simulink model "MdXX_RspOutComm1"  (R2018b)
settings: Solver=FixedStepDiscrete  StartTime=0.0  StopTime=10.0  FixedStep=0.01  RelTol=1e-3
undefined symbols (not defined in the file or in its folder): KeSMSuRspStatHldTm_Val, MdRspLocal2, SrcReqTp1
libraries: simulink x64, RspLib x32
(part 3 of 4)

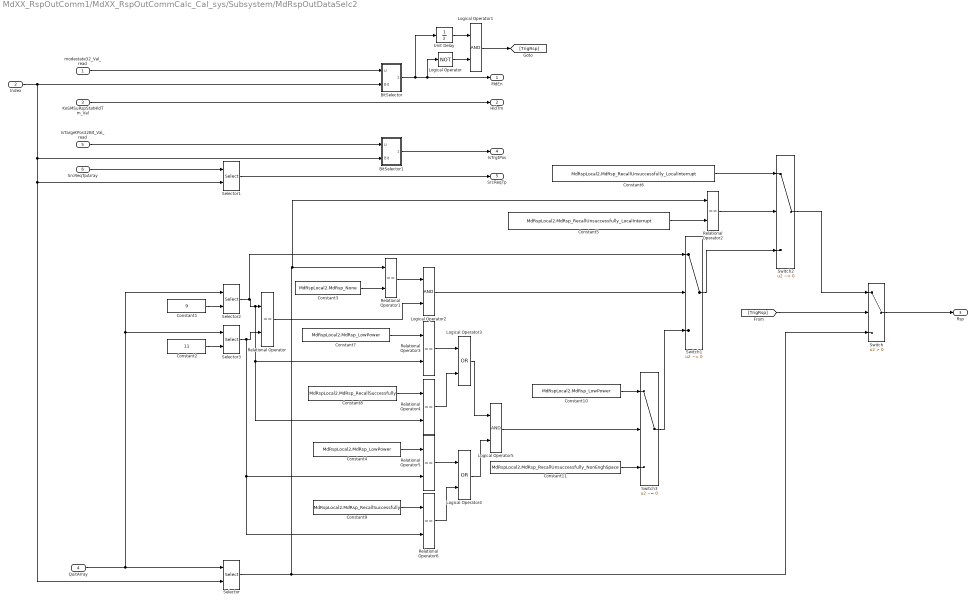
== system MdXX_RspOutComm1/MdXX_RspOutCommCalc_Cal_sys/Subsystem/MdRspOutDataSelc2 ==
  modestate32_Val_read : Inport
  Index : Inport  Port=2
  KeSMSuRspStatHldTm_Val : Inport  Port=3
  QuitArray : Inport  Port=4
  IsTargetPos32Bit_Val_read : Inport  Port=5
  SrcReqTpArray : Inport  Port=6
  BitSelector : Subsystem
  BitSelector1 : Subsystem
  Constant1 : Constant  Value=9  OutDataTypeStr=uint8
  Constant10 : Constant  Value=MdRspLocal2.MdRsp_LowPower  OutDataTypeStr=Enum: MdRspLocal2
  Constant11 : Constant  Value=MdRspLocal2.MdRsp_RecallUnsuccessfully_NonEnghSpace  OutDataTypeStr=Enum: MdRspLocal2
  Constant2 : Constant  Value=11  OutDataTypeStr=uint8
  Constant3 : Constant  Value=MdRspLocal2.MdRsp_None  OutDataTypeStr=Enum: MdRspLocal2
  Constant4 : Constant  Value=MdRspLocal2.MdRsp_LowPower  OutDataTypeStr=Enum: MdRspLocal2
  Constant5 : Constant  Value=MdRspLocal2.MdRsp_RecallUnsuccessfully_LocalInterrupt  OutDataTypeStr=Enum: MdRspLocal2
  Constant6 : Constant  Value=MdRspLocal2.MdRsp_RecallUnsuccessfully_LocalInterrupt  OutDataTypeStr=Enum: MdRspLocal2
  Constant7 : Constant  Value=MdRspLocal2.MdRsp_LowPower  OutDataTypeStr=Enum: MdRspLocal2
  Constant8 : Constant  Value=MdRspLocal2.MdRsp_RecallSuccessfully  OutDataTypeStr=Enum: MdRspLocal2
  Constant9 : Constant  Value=MdRspLocal2.MdRsp_RecallSuccessfully  OutDataTypeStr=Enum: MdRspLocal2
  Logical Operator : Logic  Operator=NOT  AllPortsSameDT=off  OutDataTypeStr=boolean
  Logical Operator1 : Logic  AllPortsSameDT=off  OutDataTypeStr=boolean
  Logical Operator2 : Logic  AllPortsSameDT=off  OutDataTypeStr=boolean
  Logical Operator3 : Logic  Operator=OR  AllPortsSameDT=off  OutDataTypeStr=boolean
  Logical Operator4 : Logic  Operator=OR  AllPortsSameDT=off  OutDataTypeStr=boolean
  Logical Operator5 : Logic  AllPortsSameDT=off  OutDataTypeStr=boolean
  Relational Operator{,1..6} (7 alike) : RelationalOperator  Operator===  OutDataTypeStr=boolean  RndMeth=Simplest
  Selector{,1..3} (4 alike) : Selector  IndexMode=Zero-based  InputPortWidth=32  IndexOptions=Index vector (port)  Indices=[1 3]  OutputSizes=1
  Switch : Switch  Criteria=u2 > Threshold
  Switch1 : Switch  Criteria=u2 ~= 0
  Switch2 : Switch  Criteria=u2 ~= 0
  Switch3 : Switch  Criteria=u2 ~= 0
  Unit Delay : UnitDelay  SampleTime=-1
  MdEn : Outport
  HldTm : Outport  Port=2
  Rsp : Outport  Port=3
  IsTrgtPos : Outport  Port=4
  SrcReqTp : Outport  Port=5
  wires:
  KeSMSuRspStatHldTm_Val/1 -> HldTm/1
  Index/1 -> BitSelector/2(Bit), Selector/2, Selector1/2, BitSelector1/2(Bit)
  Selector/1 -> Relational Operator2/1, Relational Operator1/1, Switch/3
  BitSelector/1(BitOut) -> Unit Delay/1, Logical Operator/1, MdEn/1
  modestate32_Val_read/1 -> BitSelector/1(U)
  BitSelector1/1(BitOut) -> IsTrgtPos/1
  IsTargetPos32Bit_Val_read/1 -> BitSelector1/1(U)
  QuitArray/1 -> Selector3/1, Selector2/1, Selector/1
  SrcReqTpArray/1 -> Selector1/1
  Selector1/1 -> SrcReqTp/1
  Unit Delay/1 -> Logical Operator1/1
  Logical Operator/1 -> Logical Operator1/2
  Logical Operator1/1 -> [TrigRsp]
  [TrigRsp] -> Switch/2
  Constant1/1 -> Selector2/2
  Constant2/1 -> Selector3/2
  Selector2/1 -> Switch1/1, Relational Operator/1, Relational Operator4/2, Relational Operator3/2
  Relational Operator/1 -> Logical Operator2/2
  Relational Operator1/1 -> Logical Operator2/1
  Constant3/1 -> Relational Operator1/2
  Logical Operator2/1 -> Switch1/2
  Switch/1 -> Rsp/1
  Constant5/1 -> Relational Operator2/2
  Relational Operator2/1 -> Switch2/2
  Constant6/1 -> Switch2/1
  Switch1/1 -> Switch2/3
  Switch2/1 -> Switch/1
  Switch3/1 -> Switch1/3
  Constant7/1 -> Relational Operator3/1
  Relational Operator3/1 -> Logical Operator3/1
  Relational Operator4/1 -> Logical Operator3/2
  Constant8/1 -> Relational Operator4/1
  Relational Operator5/1 -> Logical Operator4/1
  Constant4/1 -> Relational Operator5/1
  Relational Operator6/1 -> Logical Operator4/2
  Constant9/1 -> Relational Operator6/1
  Selector3/1 -> Relational Operator6/2, Relational Operator5/2, Relational Operator/2
  Logical Operator3/1 -> Logical Operator5/1
  Logical Operator4/1 -> Logical Operator5/2
  Logical Operator5/1 -> Switch3/2
  Constant10/1 -> Switch3/1
  Constant11/1 -> Switch3/3

== system MdXX_RspOutComm1/MdXX_RspOutCommCalc_Cal_sys/Subsystem/MdRspOutDataSelc20 ==
  modestate32_Val_read : Inport
  Index : Inport  Port=2
  KeSMSuRspStatHldTm_Val : Inport  Port=3
  QuitArray : Inport  Port=4
  IsTargetPos32Bit_Val_read : Inport  Port=5
  SrcReqTpArray : Inport  Port=6
  BitSelector : Subsystem
  BitSelector1 : Subsystem
  Selector : Selector  IndexMode=Zero-based  InputPortWidth=32  IndexOptions=Index vector (port)  Indices=[1 3]  OutputSizes=1
  Selector1 : Selector  IndexMode=Zero-based  InputPortWidth=32  IndexOptions=Index vector (port)  Indices=[1 3]  OutputSizes=1
  MdEn : Outport
  HldTm : Outport  Port=2
  Rsp : Outport  Port=3
  IsTrgtPos : Outport  Port=4
  SrcReqTp : Outport  Port=5
  wires:
  KeSMSuRspStatHldTm_Val/1 -> HldTm/1
  Index/1 -> BitSelector/2(Bit), Selector/2, Selector1/2, BitSelector1/2(Bit)
  Selector/1 -> Rsp/1
  BitSelector/1(BitOut) -> MdEn/1
  modestate32_Val_read/1 -> BitSelector/1(U)
  BitSelector1/1(BitOut) -> IsTrgtPos/1
  IsTargetPos32Bit_Val_read/1 -> BitSelector1/1(U)
  QuitArray/1 -> Selector/1
  SrcReqTpArray/1 -> Selector1/1
  Selector1/1 -> SrcReqTp/1

== system MdXX_RspOutComm1/MdXX_RspOutCommCalc_Cal_sys/Subsystem/MdRspOutDataSelc21 ==
  modestate32_Val_read : Inport
  Index : Inport  Port=2
  KeSMSuRspStatHldTm_Val : Inport  Port=3
  QuitArray : Inport  Port=4
  IsTargetPos32Bit_Val_read : Inport  Port=5
  SrcReqTpArray : Inport  Port=6
  BitSelector : Subsystem
  BitSelector1 : Subsystem
  Selector : Selector  IndexMode=Zero-based  InputPortWidth=32  IndexOptions=Index vector (port)  Indices=[1 3]  OutputSizes=1
  Selector1 : Selector  IndexMode=Zero-based  InputPortWidth=32  IndexOptions=Index vector (port)  Indices=[1 3]  OutputSizes=1
  MdEn : Outport
  HldTm : Outport  Port=2
  Rsp : Outport  Port=3
  IsTrgtPos : Outport  Port=4
  SrcReqTp : Outport  Port=5
  wires:
  Selector1/1 -> SrcReqTp/1
  SrcReqTpArray/1 -> Selector1/1
  QuitArray/1 -> Selector/1
  IsTargetPos32Bit_Val_read/1 -> BitSelector1/1(U)
  BitSelector1/1(BitOut) -> IsTrgtPos/1
  modestate32_Val_read/1 -> BitSelector/1(U)
  BitSelector/1(BitOut) -> MdEn/1
  Selector/1 -> Rsp/1
  Index/1 -> BitSelector1/2(Bit), Selector1/2, Selector/2, BitSelector/2(Bit)
  KeSMSuRspStatHldTm_Val/1 -> HldTm/1

== system MdXX_RspOutComm1/MdXX_RspOutCommCalc_Cal_sys/Subsystem/MdRspOutDataSelc22 ==
  modestate32_Val_read : Inport
  Index : Inport  Port=2
  KeSMSuRspStatHldTm_Val : Inport  Port=3
  QuitArray : Inport  Port=4
  IsTargetPos32Bit_Val_read : Inport  Port=5
  SrcReqTpArray : Inport  Port=6
  BitSelector : Subsystem
  BitSelector1 : Subsystem
  Selector : Selector  IndexMode=Zero-based  InputPortWidth=32  IndexOptions=Index vector (port)  Indices=[1 3]  OutputSizes=1
  Selector1 : Selector  IndexMode=Zero-based  InputPortWidth=32  IndexOptions=Index vector (port)  Indices=[1 3]  OutputSizes=1
  MdEn : Outport
  HldTm : Outport  Port=2
  Rsp : Outport  Port=3
  IsTrgtPos : Outport  Port=4
  SrcReqTp : Outport  Port=5
  wires:
  KeSMSuRspStatHldTm_Val/1 -> HldTm/1
  Index/1 -> BitSelector/2(Bit), Selector/2, Selector1/2, BitSelector1/2(Bit)
  Selector/1 -> Rsp/1
  BitSelector/1(BitOut) -> MdEn/1
  modestate32_Val_read/1 -> BitSelector/1(U)
  BitSelector1/1(BitOut) -> IsTrgtPos/1
  IsTargetPos32Bit_Val_read/1 -> BitSelector1/1(U)
  QuitArray/1 -> Selector/1
  SrcReqTpArray/1 -> Selector1/1
  Selector1/1 -> SrcReqTp/1

== system MdXX_RspOutComm1/MdXX_RspOutCommCalc_Cal_sys/Subsystem/MdRspOutDataSelc23 ==
  modestate32_Val_read : Inport
  Index : Inport  Port=2
  KeSMSuRspStatHldTm_Val : Inport  Port=3
  QuitArray : Inport  Port=4
  IsTargetPos32Bit_Val_read : Inport  Port=5
  SrcReqTpArray : Inport  Port=6
  BitSelector : Subsystem
  BitSelector1 : Subsystem
  Selector : Selector  IndexMode=Zero-based  InputPortWidth=32  IndexOptions=Index vector (port)  Indices=[1 3]  OutputSizes=1
  Selector1 : Selector  IndexMode=Zero-based  InputPortWidth=32  IndexOptions=Index vector (port)  Indices=[1 3]  OutputSizes=1
  MdEn : Outport
  HldTm : Outport  Port=2
  Rsp : Outport  Port=3
  IsTrgtPos : Outport  Port=4
  SrcReqTp : Outport  Port=5
  wires:
  Selector1/1 -> SrcReqTp/1
  SrcReqTpArray/1 -> Selector1/1
  QuitArray/1 -> Selector/1
  IsTargetPos32Bit_Val_read/1 -> BitSelector1/1(U)
  BitSelector1/1(BitOut) -> IsTrgtPos/1
  modestate32_Val_read/1 -> BitSelector/1(U)
  BitSelector/1(BitOut) -> MdEn/1
  Selector/1 -> Rsp/1
  Index/1 -> BitSelector1/2(Bit), Selector1/2, Selector/2, BitSelector/2(Bit)
  KeSMSuRspStatHldTm_Val/1 -> HldTm/1

== system MdXX_RspOutComm1/MdXX_RspOutCommCalc_Cal_sys/Subsystem/MdRspOutDataSelc24 ==
  modestate32_Val_read : Inport
  Index : Inport  Port=2
  KeSMSuRspStatHldTm_Val : Inport  Port=3
  QuitArray : Inport  Port=4
  IsTargetPos32Bit_Val_read : Inport  Port=5
  SrcReqTpArray : Inport  Port=6
  BitSelector : Subsystem
  BitSelector1 : Subsystem
  Selector : Selector  IndexMode=Zero-based  InputPortWidth=32  IndexOptions=Index vector (port)  Indices=[1 3]  OutputSizes=1
  Selector1 : Selector  IndexMode=Zero-based  InputPortWidth=32  IndexOptions=Index vector (port)  Indices=[1 3]  OutputSizes=1
  MdEn : Outport
  HldTm : Outport  Port=2
  Rsp : Outport  Port=3
  IsTrgtPos : Outport  Port=4
  SrcReqTp : Outport  Port=5
  wires:
  KeSMSuRspStatHldTm_Val/1 -> HldTm/1
  Index/1 -> BitSelector/2(Bit), Selector/2, Selector1/2, BitSelector1/2(Bit)
  Selector/1 -> Rsp/1
  BitSelector/1(BitOut) -> MdEn/1
  modestate32_Val_read/1 -> BitSelector/1(U)
  BitSelector1/1(BitOut) -> IsTrgtPos/1
  IsTargetPos32Bit_Val_read/1 -> BitSelector1/1(U)
  QuitArray/1 -> Selector/1
  SrcReqTpArray/1 -> Selector1/1
  Selector1/1 -> SrcReqTp/1

== system MdXX_RspOutComm1/MdXX_RspOutCommCalc_Cal_sys/Subsystem/MdRspOutDataSelc25 ==
  modestate32_Val_read : Inport
  Index : Inport  Port=2
  KeSMSuRspStatHldTm_Val : Inport  Port=3
  QuitArray : Inport  Port=4
  IsTargetPos32Bit_Val_read : Inport  Port=5
  SrcReqTpArray : Inport  Port=6
  BitSelector : Subsystem
  BitSelector1 : Subsystem
  Selector : Selector  IndexMode=Zero-based  InputPortWidth=32  IndexOptions=Index vector (port)  Indices=[1 3]  OutputSizes=1
  Selector1 : Selector  IndexMode=Zero-based  InputPortWidth=32  IndexOptions=Index vector (port)  Indices=[1 3]  OutputSizes=1
  MdEn : Outport
  HldTm : Outport  Port=2
  Rsp : Outport  Port=3
  IsTrgtPos : Outport  Port=4
  SrcReqTp : Outport  Port=5
  wires:
  Selector1/1 -> SrcReqTp/1
  SrcReqTpArray/1 -> Selector1/1
  QuitArray/1 -> Selector/1
  IsTargetPos32Bit_Val_read/1 -> BitSelector1/1(U)
  BitSelector1/1(BitOut) -> IsTrgtPos/1
  modestate32_Val_read/1 -> BitSelector/1(U)
  BitSelector/1(BitOut) -> MdEn/1
  Selector/1 -> Rsp/1
  Index/1 -> BitSelector1/2(Bit), Selector1/2, Selector/2, BitSelector/2(Bit)
  KeSMSuRspStatHldTm_Val/1 -> HldTm/1

== system MdXX_RspOutComm1/MdXX_RspOutCommCalc_Cal_sys/Subsystem/MdRspOutDataSelc26 ==
  modestate32_Val_read : Inport
  Index : Inport  Port=2
  KeSMSuRspStatHldTm_Val : Inport  Port=3
  QuitArray : Inport  Port=4
  IsTargetPos32Bit_Val_read : Inport  Port=5
  SrcReqTpArray : Inport  Port=6
  BitSelector : Subsystem
  BitSelector1 : Subsystem
  Selector : Selector  IndexMode=Zero-based  InputPortWidth=32  IndexOptions=Index vector (port)  Indices=[1 3]  OutputSizes=1
  Selector1 : Selector  IndexMode=Zero-based  InputPortWidth=32  IndexOptions=Index vector (port)  Indices=[1 3]  OutputSizes=1
  MdEn : Outport
  HldTm : Outport  Port=2
  Rsp : Outport  Port=3
  IsTrgtPos : Outport  Port=4
  SrcReqTp : Outport  Port=5
  wires:
  KeSMSuRspStatHldTm_Val/1 -> HldTm/1
  Index/1 -> BitSelector/2(Bit), Selector/2, Selector1/2, BitSelector1/2(Bit)
  Selector/1 -> Rsp/1
  BitSelector/1(BitOut) -> MdEn/1
  modestate32_Val_read/1 -> BitSelector/1(U)
  BitSelector1/1(BitOut) -> IsTrgtPos/1
  IsTargetPos32Bit_Val_read/1 -> BitSelector1/1(U)
  QuitArray/1 -> Selector/1
  SrcReqTpArray/1 -> Selector1/1
  Selector1/1 -> SrcReqTp/1

== system MdXX_RspOutComm1/MdXX_RspOutCommCalc_Cal_sys/Subsystem/MdRspOutDataSelc27 ==
  modestate32_Val_read : Inport
  Index : Inport  Port=2
  KeSMSuRspStatHldTm_Val : Inport  Port=3
  QuitArray : Inport  Port=4
  IsTargetPos32Bit_Val_read : Inport  Port=5
  SrcReqTpArray : Inport  Port=6
  BitSelector : Subsystem
  BitSelector1 : Subsystem
  Selector : Selector  IndexMode=Zero-based  InputPortWidth=32  IndexOptions=Index vector (port)  Indices=[1 3]  OutputSizes=1
  Selector1 : Selector  IndexMode=Zero-based  InputPortWidth=32  IndexOptions=Index vector (port)  Indices=[1 3]  OutputSizes=1
  MdEn : Outport
  HldTm : Outport  Port=2
  Rsp : Outport  Port=3
  IsTrgtPos : Outport  Port=4
  SrcReqTp : Outport  Port=5
  wires:
  Selector1/1 -> SrcReqTp/1
  SrcReqTpArray/1 -> Selector1/1
  QuitArray/1 -> Selector/1
  IsTargetPos32Bit_Val_read/1 -> BitSelector1/1(U)
  BitSelector1/1(BitOut) -> IsTrgtPos/1
  modestate32_Val_read/1 -> BitSelector/1(U)
  BitSelector/1(BitOut) -> MdEn/1
  Selector/1 -> Rsp/1
  Index/1 -> BitSelector1/2(Bit), Selector1/2, Selector/2, BitSelector/2(Bit)
  KeSMSuRspStatHldTm_Val/1 -> HldTm/1

== system MdXX_RspOutComm1/MdXX_RspOutCommCalc_Cal_sys/Subsystem/MdRspOutDataSelc28 ==
  modestate32_Val_read : Inport
  Index : Inport  Port=2
  KeSMSuRspStatHldTm_Val : Inport  Port=3
  QuitArray : Inport  Port=4
  IsTargetPos32Bit_Val_read : Inport  Port=5
  SrcReqTpArray : Inport  Port=6
  BitSelector : Subsystem
  BitSelector1 : Subsystem
  Selector : Selector  IndexMode=Zero-based  InputPortWidth=32  IndexOptions=Index vector (port)  Indices=[1 3]  OutputSizes=1
  Selector1 : Selector  IndexMode=Zero-based  InputPortWidth=32  IndexOptions=Index vector (port)  Indices=[1 3]  OutputSizes=1
  MdEn : Outport
  HldTm : Outport  Port=2
  Rsp : Outport  Port=3
  IsTrgtPos : Outport  Port=4
  SrcReqTp : Outport  Port=5
  wires:
  KeSMSuRspStatHldTm_Val/1 -> HldTm/1
  Index/1 -> BitSelector/2(Bit), Selector/2, Selector1/2, BitSelector1/2(Bit)
  Selector/1 -> Rsp/1
  BitSelector/1(BitOut) -> MdEn/1
  modestate32_Val_read/1 -> BitSelector/1(U)
  BitSelector1/1(BitOut) -> IsTrgtPos/1
  IsTargetPos32Bit_Val_read/1 -> BitSelector1/1(U)
  QuitArray/1 -> Selector/1
  SrcReqTpArray/1 -> Selector1/1
  Selector1/1 -> SrcReqTp/1

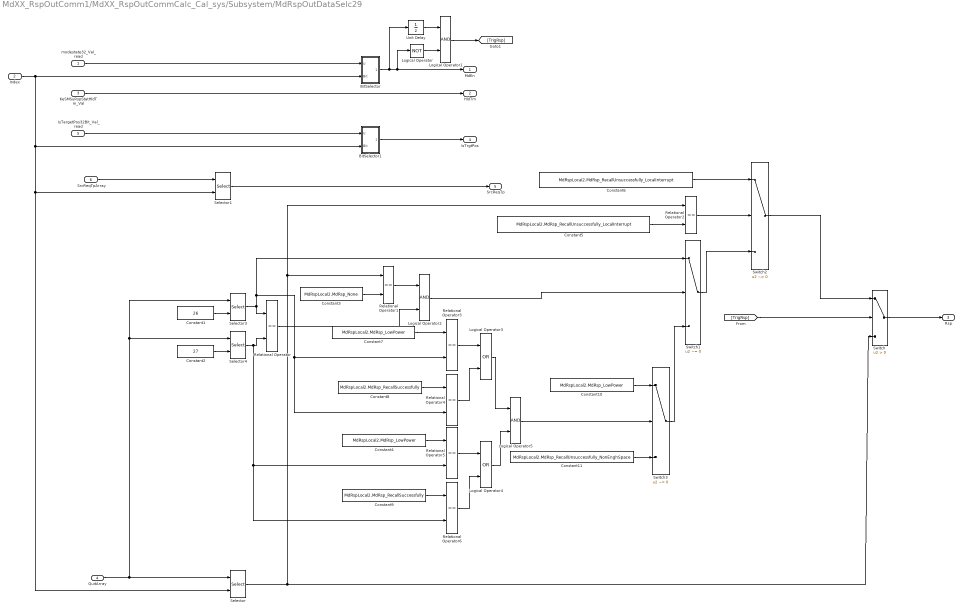
== system MdXX_RspOutComm1/MdXX_RspOutCommCalc_Cal_sys/Subsystem/MdRspOutDataSelc29 ==
  modestate32_Val_read : Inport
  Index : Inport  Port=2
  KeSMSuRspStatHldTm_Val : Inport  Port=3
  QuitArray : Inport  Port=4
  IsTargetPos32Bit_Val_read : Inport  Port=5
  SrcReqTpArray : Inport  Port=6
  BitSelector : Subsystem
  BitSelector1 : Subsystem
  Constant1 : Constant  Value=26  OutDataTypeStr=uint8
  Constant10 : Constant  Value=MdRspLocal2.MdRsp_LowPower  OutDataTypeStr=Enum: MdRspLocal2
  Constant11 : Constant  Value=MdRspLocal2.MdRsp_RecallUnsuccessfully_NonEnghSpace  OutDataTypeStr=Enum: MdRspLocal2
  Constant2 : Constant  Value=27  OutDataTypeStr=uint8
  Constant3 : Constant  Value=MdRspLocal2.MdRsp_None  OutDataTypeStr=Enum: MdRspLocal2
  Constant4 : Constant  Value=MdRspLocal2.MdRsp_LowPower  OutDataTypeStr=Enum: MdRspLocal2
  Constant5 : Constant  Value=MdRspLocal2.MdRsp_RecallUnsuccessfully_LocalInterrupt  OutDataTypeStr=Enum: MdRspLocal2
  Constant6 : Constant  Value=MdRspLocal2.MdRsp_RecallUnsuccessfully_LocalInterrupt  OutDataTypeStr=Enum: MdRspLocal2
  Constant7 : Constant  Value=MdRspLocal2.MdRsp_LowPower  OutDataTypeStr=Enum: MdRspLocal2
  Constant8 : Constant  Value=MdRspLocal2.MdRsp_RecallSuccessfully  OutDataTypeStr=Enum: MdRspLocal2
  Constant9 : Constant  Value=MdRspLocal2.MdRsp_RecallSuccessfully  OutDataTypeStr=Enum: MdRspLocal2
  Logical Operator : Logic  Operator=NOT  AllPortsSameDT=off  OutDataTypeStr=boolean
  Logical Operator1 : Logic  AllPortsSameDT=off  OutDataTypeStr=boolean
  Logical Operator2 : Logic  AllPortsSameDT=off  OutDataTypeStr=boolean
  Logical Operator3 : Logic  Operator=OR  AllPortsSameDT=off  OutDataTypeStr=boolean
  Logical Operator4 : Logic  Operator=OR  AllPortsSameDT=off  OutDataTypeStr=boolean
  Logical Operator5 : Logic  AllPortsSameDT=off  OutDataTypeStr=boolean
  Relational Operator{,1..6} (7 alike) : RelationalOperator  Operator===  OutDataTypeStr=boolean  RndMeth=Simplest
  Selector{,1,3..4} (4 alike) : Selector  IndexMode=Zero-based  InputPortWidth=32  IndexOptions=Index vector (port)  Indices=[1 3]  OutputSizes=1
  Switch : Switch  Criteria=u2 > Threshold
  Switch1 : Switch  Criteria=u2 ~= 0
  Switch2 : Switch  Criteria=u2 ~= 0
  Switch3 : Switch  Criteria=u2 ~= 0
  Unit Delay : UnitDelay  SampleTime=-1
  MdEn : Outport
  HldTm : Outport  Port=2
  Rsp : Outport  Port=3
  IsTrgtPos : Outport  Port=4
  SrcReqTp : Outport  Port=5
  wires:
  Selector1/1 -> SrcReqTp/1
  SrcReqTpArray/1 -> Selector1/1
  IsTargetPos32Bit_Val_read/1 -> BitSelector1/1(U)
  BitSelector1/1(BitOut) -> IsTrgtPos/1
  Index/1 -> Selector/2, Selector1/2, BitSelector1/2(Bit), BitSelector/2(Bit)
  KeSMSuRspStatHldTm_Val/1 -> HldTm/1
  modestate32_Val_read/1 -> BitSelector/1(U)
  BitSelector/1(BitOut) -> Unit Delay/1, Logical Operator/1, MdEn/1
  Logical Operator/1 -> Logical Operator1/2
  Logical Operator1/1 -> [TrigRsp]
  Unit Delay/1 -> Logical Operator1/1
  Switch/1 -> Rsp/1
  Relational Operator/1 -> Logical Operator2/2
  Constant1/1 -> Selector3/2
  Constant3/1 -> Relational Operator1/2
  Logical Operator2/1 -> Switch1/2
  Constant2/1 -> Selector4/2
  Relational Operator1/1 -> Logical Operator2/1
  QuitArray/1 -> Selector3/1, Selector4/1, Selector/1
  [TrigRsp] -> Switch/2
  Switch3/1 -> Switch1/3
  Constant5/1 -> Relational Operator2/2
  Selector/1 -> Relational Operator2/1, Relational Operator1/1, Switch/3
  Switch2/1 -> Switch/1
  Switch1/1 -> Switch2/3
  Relational Operator2/1 -> Switch2/2
  Constant6/1 -> Switch2/1
  Constant4/1 -> Relational Operator5/1
  Relational Operator5/1 -> Logical Operator4/1
  Relational Operator6/1 -> Logical Operator4/2
  Constant9/1 -> Relational Operator6/1
  Selector4/1 -> Relational Operator6/2, Relational Operator5/2, Relational Operator/2
  Relational Operator3/1 -> Logical Operator3/1
  Relational Operator4/1 -> Logical Operator3/2
  Constant7/1 -> Relational Operator3/1
  Logical Operator4/1 -> Logical Operator5/2
  Selector3/1 -> Relational Operator3/2, Relational Operator4/2, Switch1/1, Relational Operator/1
  Constant8/1 -> Relational Operator4/1
  Logical Operator3/1 -> Logical Operator5/1
  Constant10/1 -> Switch3/1
  Logical Operator5/1 -> Switch3/2
  Constant11/1 -> Switch3/3

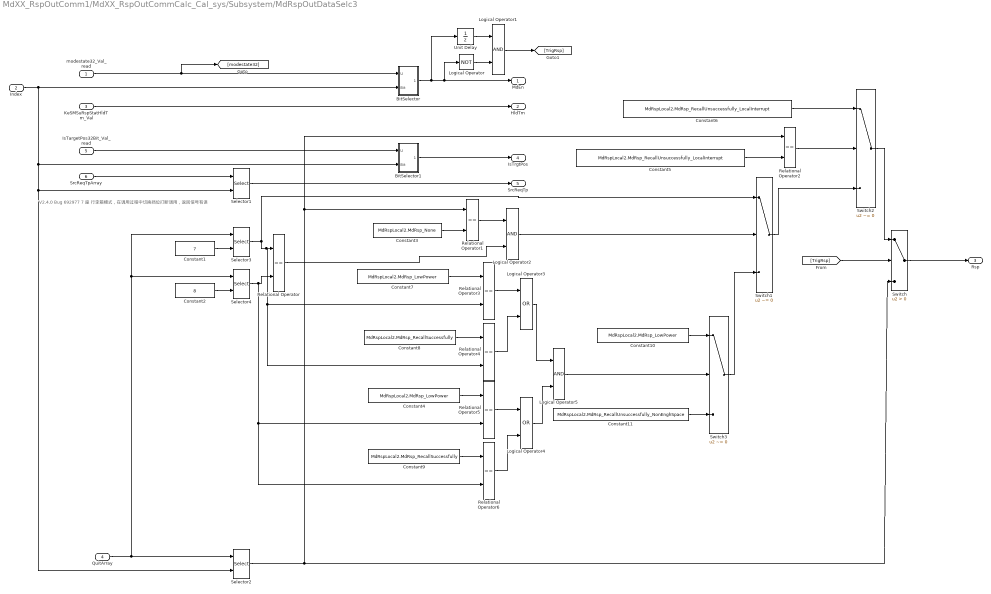
== system MdXX_RspOutComm1/MdXX_RspOutCommCalc_Cal_sys/Subsystem/MdRspOutDataSelc3 ==
  note: V2.4.0 Bug 692977 7座 行李箱模式，在调用过程中切换挡位打断调用，返回信号有误
  modestate32_Val_read : Inport
  Index : Inport  Port=2
  KeSMSuRspStatHldTm_Val : Inport  Port=3
  QuitArray : Inport  Port=4
  IsTargetPos32Bit_Val_read : Inport  Port=5
  SrcReqTpArray : Inport  Port=6
  BitSelector : Subsystem
  BitSelector1 : Subsystem
  Constant1 : Constant  Value=7  OutDataTypeStr=uint8
  Constant10 : Constant  Value=MdRspLocal2.MdRsp_LowPower  OutDataTypeStr=Enum: MdRspLocal2
  Constant11 : Constant  Value=MdRspLocal2.MdRsp_RecallUnsuccessfully_NonEnghSpace  OutDataTypeStr=Enum: MdRspLocal2
  Constant2 : Constant  Value=8  OutDataTypeStr=uint8
  Constant3 : Constant  Value=MdRspLocal2.MdRsp_None  OutDataTypeStr=Enum: MdRspLocal2
  Constant4 : Constant  Value=MdRspLocal2.MdRsp_LowPower  OutDataTypeStr=Enum: MdRspLocal2
  Constant5 : Constant  Value=MdRspLocal2.MdRsp_RecallUnsuccessfully_LocalInterrupt  OutDataTypeStr=Enum: MdRspLocal2
  Constant6 : Constant  Value=MdRspLocal2.MdRsp_RecallUnsuccessfully_LocalInterrupt  OutDataTypeStr=Enum: MdRspLocal2
  Constant7 : Constant  Value=MdRspLocal2.MdRsp_LowPower  OutDataTypeStr=Enum: MdRspLocal2
  Constant8 : Constant  Value=MdRspLocal2.MdRsp_RecallSuccessfully  OutDataTypeStr=Enum: MdRspLocal2
  Constant9 : Constant  Value=MdRspLocal2.MdRsp_RecallSuccessfully  OutDataTypeStr=Enum: MdRspLocal2
  Logical Operator : Logic  Operator=NOT  AllPortsSameDT=off  OutDataTypeStr=boolean
  Logical Operator1 : Logic  AllPortsSameDT=off  OutDataTypeStr=boolean
  Logical Operator2 : Logic  AllPortsSameDT=off  OutDataTypeStr=boolean
  Logical Operator3 : Logic  Operator=OR  AllPortsSameDT=off  OutDataTypeStr=boolean
  Logical Operator4 : Logic  Operator=OR  AllPortsSameDT=off  OutDataTypeStr=boolean
  Logical Operator5 : Logic  AllPortsSameDT=off  OutDataTypeStr=boolean
  Relational Operator{,1..6} (7 alike) : RelationalOperator  Operator===  OutDataTypeStr=boolean  RndMeth=Simplest
  Selector{1..4} (4 alike) : Selector  IndexMode=Zero-based  InputPortWidth=32  IndexOptions=Index vector (port)  Indices=[1 3]  OutputSizes=1
  Switch : Switch  Criteria=u2 > Threshold
  Switch1 : Switch  Criteria=u2 ~= 0
  Switch2 : Switch  Criteria=u2 ~= 0
  Switch3 : Switch  Criteria=u2 ~= 0
  Unit Delay : UnitDelay  SampleTime=-1
  MdEn : Outport
  HldTm : Outport  Port=2
  Rsp : Outport  Port=3
  IsTrgtPos : Outport  Port=4
  SrcReqTp : Outport  Port=5
  wires:
  Selector1/1 -> SrcReqTp/1
  SrcReqTpArray/1 -> Selector1/1
  IsTargetPos32Bit_Val_read/1 -> BitSelector1/1(U)
  BitSelector1/1(BitOut) -> IsTrgtPos/1
  modestate32_Val_read/1 -> [modestate32], BitSelector/1(U)
  KeSMSuRspStatHldTm_Val/1 -> HldTm/1
  QuitArray/1 -> Selector4/1, Selector3/1, Selector2/1
  Constant1/1 -> Selector3/2
  [TrigRsp] -> Switch/2
  Relational Operator1/1 -> Logical Operator2/1
  Constant3/1 -> Relational Operator1/2
  Logical Operator2/1 -> Switch1/2
  Relational Operator/1 -> Logical Operator2/2
  Constant2/1 -> Selector4/2
  Index/1 -> Selector2/2, Selector1/2, BitSelector1/2(Bit), BitSelector/2(Bit)
  Switch/1 -> Rsp/1
  Unit Delay/1 -> Logical Operator1/1
  Logical Operator/1 -> Logical Operator1/2
  Logical Operator1/1 -> [TrigRsp]
  BitSelector/1(BitOut) -> Unit Delay/1, Logical Operator/1, MdEn/1
  Constant5/1 -> Relational Operator2/2
  Selector2/1 -> Relational Operator2/1, Relational Operator1/1, Switch/3
  Switch2/1 -> Switch/1
  Switch1/1 -> Switch2/3
  Relational Operator2/1 -> Switch2/2
  Constant6/1 -> Switch2/1
  Constant4/1 -> Relational Operator5/1
  Relational Operator5/1 -> Logical Operator4/1
  Relational Operator6/1 -> Logical Operator4/2
  Constant9/1 -> Relational Operator6/1
  Relational Operator3/1 -> Logical Operator3/1
  Relational Operator4/1 -> Logical Operator3/2
  Switch3/1 -> Switch1/3
  Constant7/1 -> Relational Operator3/1
  Logical Operator4/1 -> Logical Operator5/2
  Constant8/1 -> Relational Operator4/1
  Logical Operator3/1 -> Logical Operator5/1
  Constant10/1 -> Switch3/1
  Selector4/1 -> Relational Operator6/2, Relational Operator5/2, Relational Operator/2
  Logical Operator5/1 -> Switch3/2
  Selector3/1 -> Switch1/1, Relational Operator4/2, Relational Operator3/2, Relational Operator/1
  Constant11/1 -> Switch3/3

== system MdXX_RspOutComm1/MdXX_RspOutCommCalc_Cal_sys/Subsystem/MdRspOutDataSelc30 ==
  modestate32_Val_read : Inport
  Index : Inport  Port=2
  KeSMSuRspStatHldTm_Val : Inport  Port=3
  QuitArray : Inport  Port=4
  IsTargetPos32Bit_Val_read : Inport  Port=5
  SrcReqTpArray : Inport  Port=6
  BitSelector : Subsystem
  BitSelector1 : Subsystem
  Selector : Selector  IndexMode=Zero-based  InputPortWidth=32  IndexOptions=Index vector (port)  Indices=[1 3]  OutputSizes=1
  Selector1 : Selector  IndexMode=Zero-based  InputPortWidth=32  IndexOptions=Index vector (port)  Indices=[1 3]  OutputSizes=1
  MdEn : Outport
  HldTm : Outport  Port=2
  Rsp : Outport  Port=3
  IsTrgtPos : Outport  Port=4
  SrcReqTp : Outport  Port=5
  wires:
  KeSMSuRspStatHldTm_Val/1 -> HldTm/1
  Index/1 -> BitSelector/2(Bit), Selector/2, Selector1/2, BitSelector1/2(Bit)
  Selector/1 -> Rsp/1
  BitSelector/1(BitOut) -> MdEn/1
  modestate32_Val_read/1 -> BitSelector/1(U)
  BitSelector1/1(BitOut) -> IsTrgtPos/1
  IsTargetPos32Bit_Val_read/1 -> BitSelector1/1(U)
  QuitArray/1 -> Selector/1
  SrcReqTpArray/1 -> Selector1/1
  Selector1/1 -> SrcReqTp/1

== system MdXX_RspOutComm1/MdXX_RspOutCommCalc_Cal_sys/Subsystem/MdRspOutDataSelc31 ==
  modestate32_Val_read : Inport
  Index : Inport  Port=2
  KeSMSuRspStatHldTm_Val : Inport  Port=3
  QuitArray : Inport  Port=4
  IsTargetPos32Bit_Val_read : Inport  Port=5
  SrcReqTpArray : Inport  Port=6
  BitSelector : Subsystem
  BitSelector1 : Subsystem
  Selector : Selector  IndexMode=Zero-based  InputPortWidth=32  IndexOptions=Index vector (port)  Indices=[1 3]  OutputSizes=1
  Selector1 : Selector  IndexMode=Zero-based  InputPortWidth=32  IndexOptions=Index vector (port)  Indices=[1 3]  OutputSizes=1
  MdEn : Outport
  HldTm : Outport  Port=2
  Rsp : Outport  Port=3
  IsTrgtPos : Outport  Port=4
  SrcReqTp : Outport  Port=5
  wires:
  Selector1/1 -> SrcReqTp/1
  SrcReqTpArray/1 -> Selector1/1
  QuitArray/1 -> Selector/1
  IsTargetPos32Bit_Val_read/1 -> BitSelector1/1(U)
  BitSelector1/1(BitOut) -> IsTrgtPos/1
  modestate32_Val_read/1 -> BitSelector/1(U)
  BitSelector/1(BitOut) -> MdEn/1
  Selector/1 -> Rsp/1
  Index/1 -> BitSelector1/2(Bit), Selector1/2, Selector/2, BitSelector/2(Bit)
  KeSMSuRspStatHldTm_Val/1 -> HldTm/1

== system MdXX_RspOutComm1/MdXX_RspOutCommCalc_Cal_sys/Subsystem/MdRspOutDataSelc32 ==
  modestate32_Val_read : Inport
  Index : Inport  Port=2
  KeSMSuRspStatHldTm_Val : Inport  Port=3
  QuitArray : Inport  Port=4
  IsTargetPos32Bit_Val_read : Inport  Port=5
  SrcReqTpArray : Inport  Port=6
  BitSelector : Subsystem
  BitSelector1 : Subsystem
  Selector : Selector  IndexMode=Zero-based  InputPortWidth=32  IndexOptions=Index vector (port)  Indices=[1 3]  OutputSizes=1
  Selector1 : Selector  IndexMode=Zero-based  InputPortWidth=32  IndexOptions=Index vector (port)  Indices=[1 3]  OutputSizes=1
  MdEn : Outport
  HldTm : Outport  Port=2
  Rsp : Outport  Port=3
  IsTrgtPos : Outport  Port=4
  SrcReqTp : Outport  Port=5
  wires:
  KeSMSuRspStatHldTm_Val/1 -> HldTm/1
  Index/1 -> BitSelector/2(Bit), Selector/2, Selector1/2, BitSelector1/2(Bit)
  Selector/1 -> Rsp/1
  BitSelector/1(BitOut) -> MdEn/1
  modestate32_Val_read/1 -> BitSelector/1(U)
  BitSelector1/1(BitOut) -> IsTrgtPos/1
  IsTargetPos32Bit_Val_read/1 -> BitSelector1/1(U)
  QuitArray/1 -> Selector/1
  SrcReqTpArray/1 -> Selector1/1
  Selector1/1 -> SrcReqTp/1

== system MdXX_RspOutComm1/MdXX_RspOutCommCalc_Cal_sys/Subsystem/MdRspOutDataSelc4 ==
  modestate32_Val_read : Inport
  Index : Inport  Port=2
  KeSMSuRspStatHldTm_Val : Inport  Port=3
  QuitArray : Inport  Port=4
  IsTargetPos32Bit_Val_read : Inport  Port=5
  SrcReqTpArray : Inport  Port=6
  BitSelector : Subsystem
  BitSelector1 : Subsystem
  Selector : Selector  IndexMode=Zero-based  InputPortWidth=32  IndexOptions=Index vector (port)  Indices=[1 3]  OutputSizes=1
  Selector1 : Selector  IndexMode=Zero-based  InputPortWidth=32  IndexOptions=Index vector (port)  Indices=[1 3]  OutputSizes=1
  MdEn : Outport
  HldTm : Outport  Port=2
  Rsp : Outport  Port=3
  IsTrgtPos : Outport  Port=4
  SrcReqTp : Outport  Port=5
  wires:
  KeSMSuRspStatHldTm_Val/1 -> HldTm/1
  Index/1 -> BitSelector/2(Bit), Selector/2, Selector1/2, BitSelector1/2(Bit)
  Selector/1 -> Rsp/1
  BitSelector/1(BitOut) -> MdEn/1
  modestate32_Val_read/1 -> BitSelector/1(U)
  BitSelector1/1(BitOut) -> IsTrgtPos/1
  IsTargetPos32Bit_Val_read/1 -> BitSelector1/1(U)
  QuitArray/1 -> Selector/1
  SrcReqTpArray/1 -> Selector1/1
  Selector1/1 -> SrcReqTp/1

== system MdXX_RspOutComm1/MdXX_RspOutCommCalc_Cal_sys/Subsystem/MdRspOutDataSelc5 ==
  modestate32_Val_read : Inport
  Index : Inport  Port=2
  KeSMSuRspStatHldTm_Val : Inport  Port=3
  QuitArray : Inport  Port=4
  IsTargetPos32Bit_Val_read : Inport  Port=5
  SrcReqTpArray : Inport  Port=6
  BitSelector : Subsystem
  BitSelector1 : Subsystem
  Selector : Selector  IndexMode=Zero-based  InputPortWidth=32  IndexOptions=Index vector (port)  Indices=[1 3]  OutputSizes=1
  Selector1 : Selector  IndexMode=Zero-based  InputPortWidth=32  IndexOptions=Index vector (port)  Indices=[1 3]  OutputSizes=1
  MdEn : Outport
  HldTm : Outport  Port=2
  Rsp : Outport  Port=3
  IsTrgtPos : Outport  Port=4
  SrcReqTp : Outport  Port=5
  wires:
  Selector1/1 -> SrcReqTp/1
  SrcReqTpArray/1 -> Selector1/1
  QuitArray/1 -> Selector/1
  IsTargetPos32Bit_Val_read/1 -> BitSelector1/1(U)
  BitSelector1/1(BitOut) -> IsTrgtPos/1
  modestate32_Val_read/1 -> BitSelector/1(U)
  BitSelector/1(BitOut) -> MdEn/1
  Selector/1 -> Rsp/1
  Index/1 -> BitSelector1/2(Bit), Selector1/2, Selector/2, BitSelector/2(Bit)
  KeSMSuRspStatHldTm_Val/1 -> HldTm/1

== system MdXX_RspOutComm1/MdXX_RspOutCommCalc_Cal_sys/Subsystem/MdRspOutDataSelc6 ==
  modestate32_Val_read : Inport
  Index : Inport  Port=2
  KeSMSuRspStatHldTm_Val : Inport  Port=3
  QuitArray : Inport  Port=4
  IsTargetPos32Bit_Val_read : Inport  Port=5
  SrcReqTpArray : Inport  Port=6
  BitSelector : Subsystem
  BitSelector1 : Subsystem
  Selector : Selector  IndexMode=Zero-based  InputPortWidth=32  IndexOptions=Index vector (port)  Indices=[1 3]  OutputSizes=1
  Selector1 : Selector  IndexMode=Zero-based  InputPortWidth=32  IndexOptions=Index vector (port)  Indices=[1 3]  OutputSizes=1
  MdEn : Outport
  HldTm : Outport  Port=2
  Rsp : Outport  Port=3
  IsTrgtPos : Outport  Port=4
  SrcReqTp : Outport  Port=5
  wires:
  KeSMSuRspStatHldTm_Val/1 -> HldTm/1
  Index/1 -> BitSelector/2(Bit), Selector/2, Selector1/2, BitSelector1/2(Bit)
  Selector/1 -> Rsp/1
  BitSelector/1(BitOut) -> MdEn/1
  modestate32_Val_read/1 -> BitSelector/1(U)
  BitSelector1/1(BitOut) -> IsTrgtPos/1
  IsTargetPos32Bit_Val_read/1 -> BitSelector1/1(U)
  QuitArray/1 -> Selector/1
  SrcReqTpArray/1 -> Selector1/1
  Selector1/1 -> SrcReqTp/1

== system MdXX_RspOutComm1/MdXX_RspOutCommCalc_Cal_sys/Subsystem/MdRspOutDataSelc7 ==
  modestate32_Val_read : Inport
  Index : Inport  Port=2
  KeSMSuRspStatHldTm_Val : Inport  Port=3
  QuitArray : Inport  Port=4
  IsTargetPos32Bit_Val_read : Inport  Port=5
  SrcReqTpArray : Inport  Port=6
  BitSelector : Subsystem
  BitSelector1 : Subsystem
  Selector : Selector  IndexMode=Zero-based  InputPortWidth=32  IndexOptions=Index vector (port)  Indices=[1 3]  OutputSizes=1
  Selector1 : Selector  IndexMode=Zero-based  InputPortWidth=32  IndexOptions=Index vector (port)  Indices=[1 3]  OutputSizes=1
  MdEn : Outport
  HldTm : Outport  Port=2
  Rsp : Outport  Port=3
  IsTrgtPos : Outport  Port=4
  SrcReqTp : Outport  Port=5
  wires:
  Selector1/1 -> SrcReqTp/1
  SrcReqTpArray/1 -> Selector1/1
  QuitArray/1 -> Selector/1
  IsTargetPos32Bit_Val_read/1 -> BitSelector1/1(U)
  BitSelector1/1(BitOut) -> IsTrgtPos/1
  modestate32_Val_read/1 -> BitSelector/1(U)
  BitSelector/1(BitOut) -> MdEn/1
  Selector/1 -> Rsp/1
  Index/1 -> BitSelector1/2(Bit), Selector1/2, Selector/2, BitSelector/2(Bit)
  KeSMSuRspStatHldTm_Val/1 -> HldTm/1

== system MdXX_RspOutComm1/MdXX_RspOutCommCalc_Cal_sys/Subsystem/MdRspOutDataSelc8 ==
  modestate32_Val_read : Inport
  Index : Inport  Port=2
  KeSMSuRspStatHldTm_Val : Inport  Port=3
  QuitArray : Inport  Port=4
  IsTargetPos32Bit_Val_read : Inport  Port=5
  SrcReqTpArray : Inport  Port=6
  BitSelector : Subsystem
  BitSelector1 : Subsystem
  Selector : Selector  IndexMode=Zero-based  InputPortWidth=32  IndexOptions=Index vector (port)  Indices=[1 3]  OutputSizes=1
  Selector1 : Selector  IndexMode=Zero-based  InputPortWidth=32  IndexOptions=Index vector (port)  Indices=[1 3]  OutputSizes=1
  MdEn : Outport
  HldTm : Outport  Port=2
  Rsp : Outport  Port=3
  IsTrgtPos : Outport  Port=4
  SrcReqTp : Outport  Port=5
  wires:
  KeSMSuRspStatHldTm_Val/1 -> HldTm/1
  Index/1 -> BitSelector/2(Bit), Selector/2, Selector1/2, BitSelector1/2(Bit)
  Selector/1 -> Rsp/1
  BitSelector/1(BitOut) -> MdEn/1
  modestate32_Val_read/1 -> BitSelector/1(U)
  BitSelector1/1(BitOut) -> IsTrgtPos/1
  IsTargetPos32Bit_Val_read/1 -> BitSelector1/1(U)
  QuitArray/1 -> Selector/1
  SrcReqTpArray/1 -> Selector1/1
  Selector1/1 -> SrcReqTp/1

== system MdXX_RspOutComm1/MdXX_RspOutCommCalc_Cal_sys/Subsystem/MdRspOutDataSelc9 ==
  modestate32_Val_read : Inport
  Index : Inport  Port=2
  KeSMSuRspStatHldTm_Val : Inport  Port=3
  QuitArray : Inport  Port=4
  IsTargetPos32Bit_Val_read : Inport  Port=5
  SrcReqTpArray : Inport  Port=6
  BitSelector : Subsystem
  BitSelector1 : Subsystem
  Selector : Selector  IndexMode=Zero-based  InputPortWidth=32  IndexOptions=Index vector (port)  Indices=[1 3]  OutputSizes=1
  Selector1 : Selector  IndexMode=Zero-based  InputPortWidth=32  IndexOptions=Index vector (port)  Indices=[1 3]  OutputSizes=1
  MdEn : Outport
  HldTm : Outport  Port=2
  Rsp : Outport  Port=3
  IsTrgtPos : Outport  Port=4
  SrcReqTp : Outport  Port=5
  wires:
  Selector1/1 -> SrcReqTp/1
  SrcReqTpArray/1 -> Selector1/1
  QuitArray/1 -> Selector/1
  IsTargetPos32Bit_Val_read/1 -> BitSelector1/1(U)
  BitSelector1/1(BitOut) -> IsTrgtPos/1
  modestate32_Val_read/1 -> BitSelector/1(U)
  BitSelector/1(BitOut) -> MdEn/1
  Selector/1 -> Rsp/1
  Index/1 -> BitSelector1/2(Bit), Selector1/2, Selector/2, BitSelector/2(Bit)
  KeSMSuRspStatHldTm_Val/1 -> HldTm/1

== system MdXX_RspOutComm1/MdXX_RspOutCommCalc_Cal_sys/Subsystem/MdRspOutDataSelc1/BitSelector ==
  U : Inport
  Bit : Inport  Port=2
  Bitwise Operator : simulink/Logic and Bit Operations/Bitwise Operator  logicop=AND  UseBitMask=off  NumInputPorts=2  BitMask=bin2dec('11011001')  BitMaskRealWorld=Stored Integer
  Constant2 : Constant  OutDataTypeStr=uint32
  Constant4 : Constant  Value=0  OutDataTypeStr=uint32
  Relational Operator : RelationalOperator  Operator=>  OutDataTypeStr=boolean  RndMeth=Simplest
  Shift Arithmetic : ArithShift  BitShiftNumberSource=Input port  BitShiftNumber=8  BitShiftDirection=Left
      settings: InputPortMap=u0,p1
  BitOut : Outport
  wires:
  Relational Operator/1 -> BitOut/1
  Constant4/1 -> Relational Operator/2
  Constant2/1 -> Shift Arithmetic/1
  Bitwise Operator/1 -> Relational Operator/1
  U/1 -> Bitwise Operator/1
  Shift Arithmetic/1 -> Bitwise Operator/2
  Bit/1 -> Shift Arithmetic/2

== system MdXX_RspOutComm1/MdXX_RspOutCommCalc_Cal_sys/Subsystem/MdRspOutDataSelc1/BitSelector1 ==
  U : Inport
  Bit : Inport  Port=2
  Bitwise Operator : simulink/Logic and Bit Operations/Bitwise Operator  logicop=AND  UseBitMask=off  NumInputPorts=2  BitMask=bin2dec('11011001')  BitMaskRealWorld=Stored Integer
  Constant2 : Constant  OutDataTypeStr=uint32
  Constant4 : Constant  Value=0  OutDataTypeStr=uint32
  Relational Operator : RelationalOperator  Operator=>  OutDataTypeStr=boolean  RndMeth=Simplest
  Shift Arithmetic : ArithShift  BitShiftNumberSource=Input port  BitShiftNumber=8  BitShiftDirection=Left
      settings: InputPortMap=u0,p1
  BitOut : Outport
  wires:
  Bit/1 -> Shift Arithmetic/2
  Shift Arithmetic/1 -> Bitwise Operator/2
  U/1 -> Bitwise Operator/1
  Bitwise Operator/1 -> Relational Operator/1
  Constant2/1 -> Shift Arithmetic/1
  Constant4/1 -> Relational Operator/2
  Relational Operator/1 -> BitOut/1

== system MdXX_RspOutComm1/MdXX_RspOutCommCalc_Cal_sys/Subsystem/MdRspOutDataSelc10/BitSelector ==
  U : Inport
  Bit : Inport  Port=2
  Bitwise Operator : simulink/Logic and Bit Operations/Bitwise Operator  logicop=AND  UseBitMask=off  NumInputPorts=2  BitMask=bin2dec('11011001')  BitMaskRealWorld=Stored Integer
  Constant2 : Constant  OutDataTypeStr=uint32
  Constant4 : Constant  Value=0  OutDataTypeStr=uint32
  Relational Operator : RelationalOperator  Operator=>  OutDataTypeStr=boolean  RndMeth=Simplest
  Shift Arithmetic : ArithShift  BitShiftNumberSource=Input port  BitShiftNumber=8  BitShiftDirection=Left
      settings: InputPortMap=u0,p1
  BitOut : Outport
  wires:
  Bit/1 -> Shift Arithmetic/2
  Shift Arithmetic/1 -> Bitwise Operator/2
  U/1 -> Bitwise Operator/1
  Bitwise Operator/1 -> Relational Operator/1
  Constant2/1 -> Shift Arithmetic/1
  Constant4/1 -> Relational Operator/2
  Relational Operator/1 -> BitOut/1

== system MdXX_RspOutComm1/MdXX_RspOutCommCalc_Cal_sys/Subsystem/MdRspOutDataSelc10/BitSelector1 ==
  U : Inport
  Bit : Inport  Port=2
  Bitwise Operator : simulink/Logic and Bit Operations/Bitwise Operator  logicop=AND  UseBitMask=off  NumInputPorts=2  BitMask=bin2dec('11011001')  BitMaskRealWorld=Stored Integer
  Constant2 : Constant  OutDataTypeStr=uint32
  Constant4 : Constant  Value=0  OutDataTypeStr=uint32
  Relational Operator : RelationalOperator  Operator=>  OutDataTypeStr=boolean  RndMeth=Simplest
  Shift Arithmetic : ArithShift  BitShiftNumberSource=Input port  BitShiftNumber=8  BitShiftDirection=Left
      settings: InputPortMap=u0,p1
  BitOut : Outport
  wires:
  Relational Operator/1 -> BitOut/1
  Constant4/1 -> Relational Operator/2
  Constant2/1 -> Shift Arithmetic/1
  Bitwise Operator/1 -> Relational Operator/1
  U/1 -> Bitwise Operator/1
  Shift Arithmetic/1 -> Bitwise Operator/2
  Bit/1 -> Shift Arithmetic/2

== system MdXX_RspOutComm1/MdXX_RspOutCommCalc_Cal_sys/Subsystem/MdRspOutDataSelc11/BitSelector ==
  U : Inport
  Bit : Inport  Port=2
  Bitwise Operator : simulink/Logic and Bit Operations/Bitwise Operator  logicop=AND  UseBitMask=off  NumInputPorts=2  BitMask=bin2dec('11011001')  BitMaskRealWorld=Stored Integer
  Constant2 : Constant  OutDataTypeStr=uint32
  Constant4 : Constant  Value=0  OutDataTypeStr=uint32
  Relational Operator : RelationalOperator  Operator=>  OutDataTypeStr=boolean  RndMeth=Simplest
  Shift Arithmetic : ArithShift  BitShiftNumberSource=Input port  BitShiftNumber=8  BitShiftDirection=Left
      settings: InputPortMap=u0,p1
  BitOut : Outport
  wires:
  Relational Operator/1 -> BitOut/1
  Constant4/1 -> Relational Operator/2
  Constant2/1 -> Shift Arithmetic/1
  Bitwise Operator/1 -> Relational Operator/1
  U/1 -> Bitwise Operator/1
  Shift Arithmetic/1 -> Bitwise Operator/2
  Bit/1 -> Shift Arithmetic/2

== system MdXX_RspOutComm1/MdXX_RspOutCommCalc_Cal_sys/Subsystem/MdRspOutDataSelc11/BitSelector1 ==
  U : Inport
  Bit : Inport  Port=2
  Bitwise Operator : simulink/Logic and Bit Operations/Bitwise Operator  logicop=AND  UseBitMask=off  NumInputPorts=2  BitMask=bin2dec('11011001')  BitMaskRealWorld=Stored Integer
  Constant2 : Constant  OutDataTypeStr=uint32
  Constant4 : Constant  Value=0  OutDataTypeStr=uint32
  Relational Operator : RelationalOperator  Operator=>  OutDataTypeStr=boolean  RndMeth=Simplest
  Shift Arithmetic : ArithShift  BitShiftNumberSource=Input port  BitShiftNumber=8  BitShiftDirection=Left
      settings: InputPortMap=u0,p1
  BitOut : Outport
  wires:
  Bit/1 -> Shift Arithmetic/2
  Shift Arithmetic/1 -> Bitwise Operator/2
  U/1 -> Bitwise Operator/1
  Bitwise Operator/1 -> Relational Operator/1
  Constant2/1 -> Shift Arithmetic/1
  Constant4/1 -> Relational Operator/2
  Relational Operator/1 -> BitOut/1

== system MdXX_RspOutComm1/MdXX_RspOutCommCalc_Cal_sys/Subsystem/MdRspOutDataSelc12/BitSelector ==
  U : Inport
  Bit : Inport  Port=2
  Bitwise Operator : simulink/Logic and Bit Operations/Bitwise Operator  logicop=AND  UseBitMask=off  NumInputPorts=2  BitMask=bin2dec('11011001')  BitMaskRealWorld=Stored Integer
  Constant2 : Constant  OutDataTypeStr=uint32
  Constant4 : Constant  Value=0  OutDataTypeStr=uint32
  Relational Operator : RelationalOperator  Operator=>  OutDataTypeStr=boolean  RndMeth=Simplest
  Shift Arithmetic : ArithShift  BitShiftNumberSource=Input port  BitShiftNumber=8  BitShiftDirection=Left
      settings: InputPortMap=u0,p1
  BitOut : Outport
  wires:
  Bit/1 -> Shift Arithmetic/2
  Shift Arithmetic/1 -> Bitwise Operator/2
  U/1 -> Bitwise Operator/1
  Bitwise Operator/1 -> Relational Operator/1
  Constant2/1 -> Shift Arithmetic/1
  Constant4/1 -> Relational Operator/2
  Relational Operator/1 -> BitOut/1

== system MdXX_RspOutComm1/MdXX_RspOutCommCalc_Cal_sys/Subsystem/MdRspOutDataSelc12/BitSelector1 ==
  U : Inport
  Bit : Inport  Port=2
  Bitwise Operator : simulink/Logic and Bit Operations/Bitwise Operator  logicop=AND  UseBitMask=off  NumInputPorts=2  BitMask=bin2dec('11011001')  BitMaskRealWorld=Stored Integer
  Constant2 : Constant  OutDataTypeStr=uint32
  Constant4 : Constant  Value=0  OutDataTypeStr=uint32
  Relational Operator : RelationalOperator  Operator=>  OutDataTypeStr=boolean  RndMeth=Simplest
  Shift Arithmetic : ArithShift  BitShiftNumberSource=Input port  BitShiftNumber=8  BitShiftDirection=Left
      settings: InputPortMap=u0,p1
  BitOut : Outport
  wires:
  Relational Operator/1 -> BitOut/1
  Constant4/1 -> Relational Operator/2
  Constant2/1 -> Shift Arithmetic/1
  Bitwise Operator/1 -> Relational Operator/1
  U/1 -> Bitwise Operator/1
  Shift Arithmetic/1 -> Bitwise Operator/2
  Bit/1 -> Shift Arithmetic/2

== system MdXX_RspOutComm1/MdXX_RspOutCommCalc_Cal_sys/Subsystem/MdRspOutDataSelc13/BitSelector ==
  U : Inport
  Bit : Inport  Port=2
  Bitwise Operator : simulink/Logic and Bit Operations/Bitwise Operator  logicop=AND  UseBitMask=off  NumInputPorts=2  BitMask=bin2dec('11011001')  BitMaskRealWorld=Stored Integer
  Constant2 : Constant  OutDataTypeStr=uint32
  Constant4 : Constant  Value=0  OutDataTypeStr=uint32
  Relational Operator : RelationalOperator  Operator=>  OutDataTypeStr=boolean  RndMeth=Simplest
  Shift Arithmetic : ArithShift  BitShiftNumberSource=Input port  BitShiftNumber=8  BitShiftDirection=Left
      settings: InputPortMap=u0,p1
  BitOut : Outport
  wires:
  Relational Operator/1 -> BitOut/1
  Constant4/1 -> Relational Operator/2
  Constant2/1 -> Shift Arithmetic/1
  Bitwise Operator/1 -> Relational Operator/1
  U/1 -> Bitwise Operator/1
  Shift Arithmetic/1 -> Bitwise Operator/2
  Bit/1 -> Shift Arithmetic/2

== system MdXX_RspOutComm1/MdXX_RspOutCommCalc_Cal_sys/Subsystem/MdRspOutDataSelc13/BitSelector1 ==
  U : Inport
  Bit : Inport  Port=2
  Bitwise Operator : simulink/Logic and Bit Operations/Bitwise Operator  logicop=AND  UseBitMask=off  NumInputPorts=2  BitMask=bin2dec('11011001')  BitMaskRealWorld=Stored Integer
  Constant2 : Constant  OutDataTypeStr=uint32
  Constant4 : Constant  Value=0  OutDataTypeStr=uint32
  Relational Operator : RelationalOperator  Operator=>  OutDataTypeStr=boolean  RndMeth=Simplest
  Shift Arithmetic : ArithShift  BitShiftNumberSource=Input port  BitShiftNumber=8  BitShiftDirection=Left
      settings: InputPortMap=u0,p1
  BitOut : Outport
  wires:
  Bit/1 -> Shift Arithmetic/2
  Shift Arithmetic/1 -> Bitwise Operator/2
  U/1 -> Bitwise Operator/1
  Bitwise Operator/1 -> Relational Operator/1
  Constant2/1 -> Shift Arithmetic/1
  Constant4/1 -> Relational Operator/2
  Relational Operator/1 -> BitOut/1

== system MdXX_RspOutComm1/MdXX_RspOutCommCalc_Cal_sys/Subsystem/MdRspOutDataSelc14/BitSelector ==
  U : Inport
  Bit : Inport  Port=2
  Bitwise Operator : simulink/Logic and Bit Operations/Bitwise Operator  logicop=AND  UseBitMask=off  NumInputPorts=2  BitMask=bin2dec('11011001')  BitMaskRealWorld=Stored Integer
  Constant2 : Constant  OutDataTypeStr=uint32
  Constant4 : Constant  Value=0  OutDataTypeStr=uint32
  Relational Operator : RelationalOperator  Operator=>  OutDataTypeStr=boolean  RndMeth=Simplest
  Shift Arithmetic : ArithShift  BitShiftNumberSource=Input port  BitShiftNumber=8  BitShiftDirection=Left
      settings: InputPortMap=u0,p1
  BitOut : Outport
  wires:
  Bit/1 -> Shift Arithmetic/2
  Shift Arithmetic/1 -> Bitwise Operator/2
  U/1 -> Bitwise Operator/1
  Bitwise Operator/1 -> Relational Operator/1
  Constant2/1 -> Shift Arithmetic/1
  Constant4/1 -> Relational Operator/2
  Relational Operator/1 -> BitOut/1

== system MdXX_RspOutComm1/MdXX_RspOutCommCalc_Cal_sys/Subsystem/MdRspOutDataSelc14/BitSelector1 ==
  U : Inport
  Bit : Inport  Port=2
  Bitwise Operator : simulink/Logic and Bit Operations/Bitwise Operator  logicop=AND  UseBitMask=off  NumInputPorts=2  BitMask=bin2dec('11011001')  BitMaskRealWorld=Stored Integer
  Constant2 : Constant  OutDataTypeStr=uint32
  Constant4 : Constant  Value=0  OutDataTypeStr=uint32
  Relational Operator : RelationalOperator  Operator=>  OutDataTypeStr=boolean  RndMeth=Simplest
  Shift Arithmetic : ArithShift  BitShiftNumberSource=Input port  BitShiftNumber=8  BitShiftDirection=Left
      settings: InputPortMap=u0,p1
  BitOut : Outport
  wires:
  Relational Operator/1 -> BitOut/1
  Constant4/1 -> Relational Operator/2
  Constant2/1 -> Shift Arithmetic/1
  Bitwise Operator/1 -> Relational Operator/1
  U/1 -> Bitwise Operator/1
  Shift Arithmetic/1 -> Bitwise Operator/2
  Bit/1 -> Shift Arithmetic/2

== system MdXX_RspOutComm1/MdXX_RspOutCommCalc_Cal_sys/Subsystem/MdRspOutDataSelc15/BitSelector ==
  U : Inport
  Bit : Inport  Port=2
  Bitwise Operator : simulink/Logic and Bit Operations/Bitwise Operator  logicop=AND  UseBitMask=off  NumInputPorts=2  BitMask=bin2dec('11011001')  BitMaskRealWorld=Stored Integer
  Constant2 : Constant  OutDataTypeStr=uint32
  Constant4 : Constant  Value=0  OutDataTypeStr=uint32
  Relational Operator : RelationalOperator  Operator=>  OutDataTypeStr=boolean  RndMeth=Simplest
  Shift Arithmetic : ArithShift  BitShiftNumberSource=Input port  BitShiftNumber=8  BitShiftDirection=Left
      settings: InputPortMap=u0,p1
  BitOut : Outport
  wires:
  Relational Operator/1 -> BitOut/1
  Constant4/1 -> Relational Operator/2
  Constant2/1 -> Shift Arithmetic/1
  Bitwise Operator/1 -> Relational Operator/1
  U/1 -> Bitwise Operator/1
  Shift Arithmetic/1 -> Bitwise Operator/2
  Bit/1 -> Shift Arithmetic/2

== system MdXX_RspOutComm1/MdXX_RspOutCommCalc_Cal_sys/Subsystem/MdRspOutDataSelc15/BitSelector1 ==
  U : Inport
  Bit : Inport  Port=2
  Bitwise Operator : simulink/Logic and Bit Operations/Bitwise Operator  logicop=AND  UseBitMask=off  NumInputPorts=2  BitMask=bin2dec('11011001')  BitMaskRealWorld=Stored Integer
  Constant2 : Constant  OutDataTypeStr=uint32
  Constant4 : Constant  Value=0  OutDataTypeStr=uint32
  Relational Operator : RelationalOperator  Operator=>  OutDataTypeStr=boolean  RndMeth=Simplest
  Shift Arithmetic : ArithShift  BitShiftNumberSource=Input port  BitShiftNumber=8  BitShiftDirection=Left
      settings: InputPortMap=u0,p1
  BitOut : Outport
  wires:
  Bit/1 -> Shift Arithmetic/2
  Shift Arithmetic/1 -> Bitwise Operator/2
  U/1 -> Bitwise Operator/1
  Bitwise Operator/1 -> Relational Operator/1
  Constant2/1 -> Shift Arithmetic/1
  Constant4/1 -> Relational Operator/2
  Relational Operator/1 -> BitOut/1

== system MdXX_RspOutComm1/MdXX_RspOutCommCalc_Cal_sys/Subsystem/MdRspOutDataSelc16/BitSelector ==
  U : Inport
  Bit : Inport  Port=2
  Bitwise Operator : simulink/Logic and Bit Operations/Bitwise Operator  logicop=AND  UseBitMask=off  NumInputPorts=2  BitMask=bin2dec('11011001')  BitMaskRealWorld=Stored Integer
  Constant2 : Constant  OutDataTypeStr=uint32
  Constant4 : Constant  Value=0  OutDataTypeStr=uint32
  Relational Operator : RelationalOperator  Operator=>  OutDataTypeStr=boolean  RndMeth=Simplest
  Shift Arithmetic : ArithShift  BitShiftNumberSource=Input port  BitShiftNumber=8  BitShiftDirection=Left
      settings: InputPortMap=u0,p1
  BitOut : Outport
  wires:
  Bit/1 -> Shift Arithmetic/2
  Shift Arithmetic/1 -> Bitwise Operator/2
  U/1 -> Bitwise Operator/1
  Bitwise Operator/1 -> Relational Operator/1
  Constant2/1 -> Shift Arithmetic/1
  Constant4/1 -> Relational Operator/2
  Relational Operator/1 -> BitOut/1

== system MdXX_RspOutComm1/MdXX_RspOutCommCalc_Cal_sys/Subsystem/MdRspOutDataSelc16/BitSelector1 ==
  U : Inport
  Bit : Inport  Port=2
  Bitwise Operator : simulink/Logic and Bit Operations/Bitwise Operator  logicop=AND  UseBitMask=off  NumInputPorts=2  BitMask=bin2dec('11011001')  BitMaskRealWorld=Stored Integer
  Constant2 : Constant  OutDataTypeStr=uint32
  Constant4 : Constant  Value=0  OutDataTypeStr=uint32
  Relational Operator : RelationalOperator  Operator=>  OutDataTypeStr=boolean  RndMeth=Simplest
  Shift Arithmetic : ArithShift  BitShiftNumberSource=Input port  BitShiftNumber=8  BitShiftDirection=Left
      settings: InputPortMap=u0,p1
  BitOut : Outport
  wires:
  Relational Operator/1 -> BitOut/1
  Constant4/1 -> Relational Operator/2
  Constant2/1 -> Shift Arithmetic/1
  Bitwise Operator/1 -> Relational Operator/1
  U/1 -> Bitwise Operator/1
  Shift Arithmetic/1 -> Bitwise Operator/2
  Bit/1 -> Shift Arithmetic/2

== system MdXX_RspOutComm1/MdXX_RspOutCommCalc_Cal_sys/Subsystem/MdRspOutDataSelc17/BitSelector ==
  U : Inport
  Bit : Inport  Port=2
  Bitwise Operator : simulink/Logic and Bit Operations/Bitwise Operator  logicop=AND  UseBitMask=off  NumInputPorts=2  BitMask=bin2dec('11011001')  BitMaskRealWorld=Stored Integer
  Constant2 : Constant  OutDataTypeStr=uint32
  Constant4 : Constant  Value=0  OutDataTypeStr=uint32
  Relational Operator : RelationalOperator  Operator=>  OutDataTypeStr=boolean  RndMeth=Simplest
  Shift Arithmetic : ArithShift  BitShiftNumberSource=Input port  BitShiftNumber=8  BitShiftDirection=Left
      settings: InputPortMap=u0,p1
  BitOut : Outport
  wires:
  Relational Operator/1 -> BitOut/1
  Constant4/1 -> Relational Operator/2
  Constant2/1 -> Shift Arithmetic/1
  Bitwise Operator/1 -> Relational Operator/1
  U/1 -> Bitwise Operator/1
  Shift Arithmetic/1 -> Bitwise Operator/2
  Bit/1 -> Shift Arithmetic/2
